simulink model "Aufgabe2_Pendulum"  (R2013a)
settings: Solver=ode45  StartTime=0.0  StopTime=10.0  RelTol=1e-3
libraries: vrlib x2
settings Model: Creator=Erwin  LastModifiedBy=Erwin

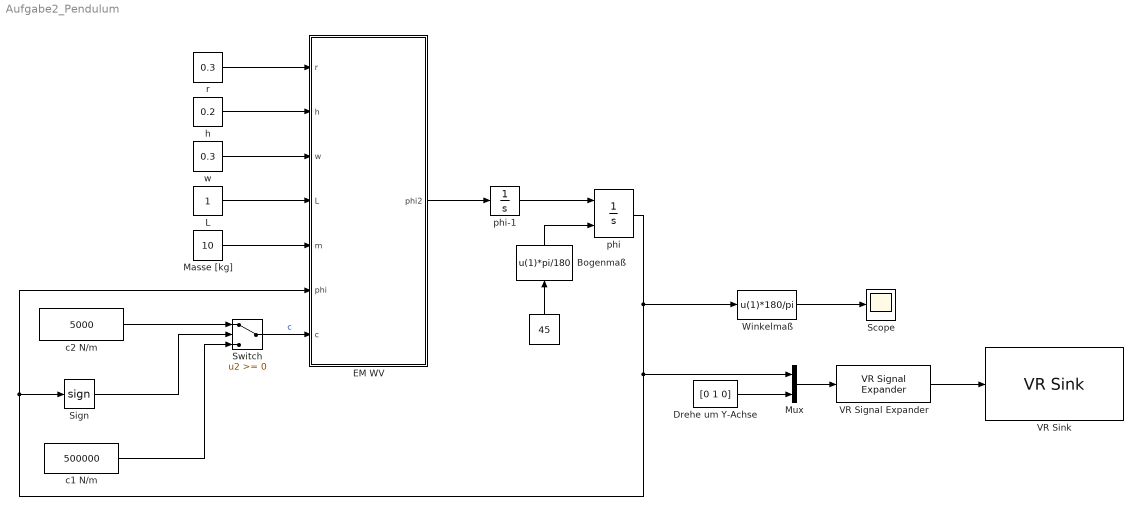
== system Aufgabe2_Pendulum ==
  " " : Constant  Value=45
  Bogenmaß : Fcn  Expr=u(1)*pi/180
  Drehe um Y-Achse : Constant  Value=[0 1 0]
  EM WV : MATLAB Function  TreatAsAtomicUnit=on
  L : Constant
  Masse [kg] : Constant  Value=10
  Mux : Mux  Inputs=2
  Scope : Scope
      settings: YMin=-45
  Sign : Signum
  Switch : Switch
  VR Signal Expander : vrlib/VR Signal Expander  outwidth=4  outidx=[4 1 2 3]
  VR Sink : vrlib/VR Sink  InstantiateOnLoad=on  SampleTime=0.005  ViewEnable=on  RemoteChange=off  RemoteView=off  FieldsWritten=Seiltrommel.rotation.4.1.1.double  WorldFileName=C:\Users\Erwin\Dropbox\Master\Module\MD\Aufgaben\SS2015\Aufgaben von Meisel\Versuch_2\CrazyPendlm.wrl  AutoView=off  VideoDimensions=[]  AllowVariableSize=off  FigureProperties="{'Position', 'Name', 'Viewpoint', 'CameraBound', 'CameraDirection', 'CameraPosition', 'CameraUpVector', 'ZoomFactor', 'Antialiasing', 'Headlight', 'Lighting', 'NavPanel', 'StatusBar', 'ToolBar', 'Textures', 'Transparency', 'Wireframe', 'NavZones', 'NavMode', 'NavSpeed', 'Record2DCompressMethod', 'Record2DCompressQuality', 'Record2D', 'Record2DFileName', 'Record2DFPS'; [6.7700000000000000e+02   4.5500000000000000e+02   5.7600000000000000e+02   3.8000000000000000e+02], '', '', 'on', [-8.8155813548629247e-01   4.0433997304721032e-02  -4.7034066974895922e-01], [3.1410759078128292e-02   0.0000000000000000e+00   4.0004934396342682e+00], [2.1818837589458722e-02   9.9875026039496628e-01   4.4965049618920026e-02], [1.0000000000000000e+00], 'on', 'on', 'on', 'none', 'on', 'on', 'on', 'on', 'off', 'off', 'walk', 'normal', 'auto', [7.5000000000000000e+01], 'off', '%f_anim_%n.avi', [1.5000000000000000e+01]}"
  Winkelmaß : Fcn  Expr=u(1)*180/pi
  c1 N/m : Constant  Value=500000
  c2 N/m : Constant  Value=5000
  h : Constant  Value=0.2
  phi : Integrator  InitialConditionSource=external
  phi-1 : Integrator
  r : Constant  Value=0.3
  w : Constant  Value=0.3
  wires:
  Drehe um Y-Achse/1 -> Mux/2
  Mux/1 -> VR Signal Expander/1
  Bogenmaß/1 -> phi/2
  " "/1 -> Bogenmaß/1
  c1 N/m/1 -> Switch/3
  c2 N/m/1 -> Switch/1
  phi/1 -> EM WV/6(phi), Sign/1, Mux/1, Winkelmaß/1
  Sign/1 -> Switch/2
  phi-1/1 -> phi/1
  Masse [kg]/1 -> EM WV/5(m)
  L/1 -> EM WV/4(L)
  w/1 -> EM WV/3(w)
  h/1 -> EM WV/2(h)
  r/1 -> EM WV/1(r)
  EM WV/1(phi2) -> phi-1/1
  Switch/1 -> EM WV/7(c)  "c"
  Winkelmaß/1 -> Scope/1
  VR Signal Expander/1 -> VR Sink/1

== matlab function Aufgabe2_Pendulum/EM WV ==
  data: r input; h input; w input; L input; m input; phi input; phi2 output; c input
function phi2 = Winkelgeschwindigkeit(r,h,w,L,m,phi,c)

g = 9.8;
M1 = m*g*sin(phi)*(L+h/2);        
M2 = -phi*c*r^2;
J = (1/12*(h^2+w^2) + (L+h/2)^2)*m;
phi2 = (M1+M2)/J;
